simulink subsystem "Current_regulator"  (R2024b)
settings: Solver=VariableStepAuto  StartTime=0.0  StopTime=10.0  RelTol=1e-3
undefined symbols (not defined in the file): CurrentKi, CurrentKp, Ts0
libraries: simulink x1
settings Model: DataDictionary=RectData.sldd  EnableAccessToBaseWorkspace=off  Creator=sgade  LastModifiedBy=sgade

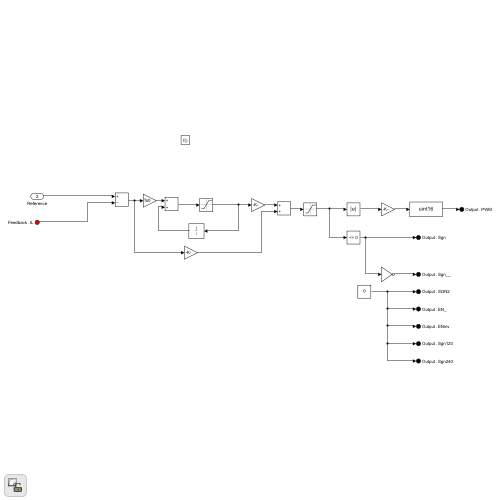
[thumbnail: Simulink's stored preview of the top-level diagram]
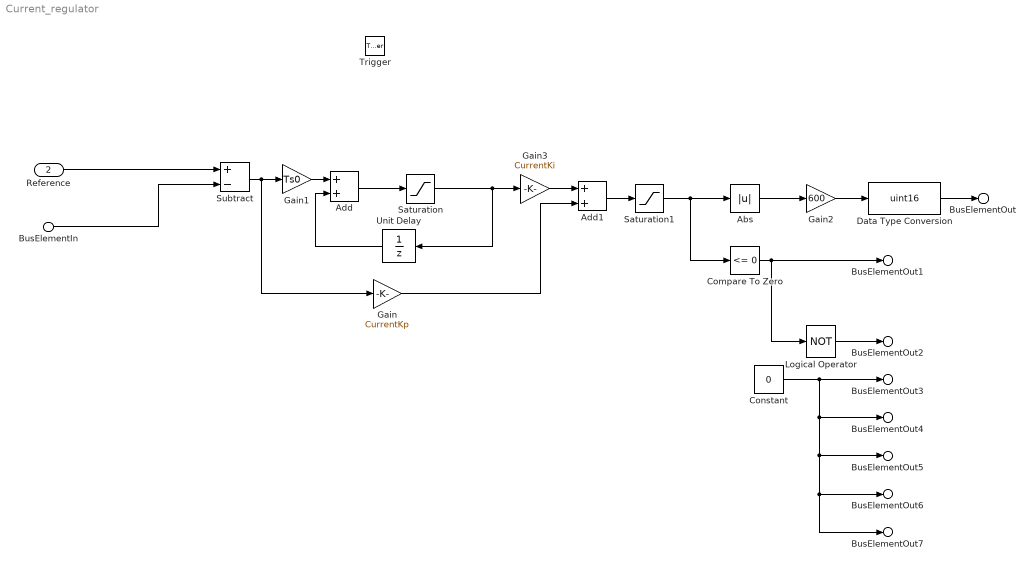
== system Current_regulator ==
  BusElementIn : Inport  PortName=Feedback  Element=IL
  Reference : Inport  Port=2
  Trigger : TriggerPort  TriggerType=function-call  VariantControl=(inherit)  PortDimensions=1
  Abs : Abs  SaturateOnIntegerOverflow=off
  Add : Sum
  Add1 : Sum
  Compare To Zero : simulink/Logic and Bit Operations/Compare To Zero  relop=<=  OutDataTypeStr=boolean
  Constant : Constant  Value=0  OutDataTypeStr=boolean  SampleTime=-1
  Data Type Conversion : DataTypeConversion  OutDataTypeStr=uint16  SaturateOnIntegerOverflow=off  RndMeth=Floor
  Gain : Gain  Gain=CurrentKp  OutDataTypeStr=single
  Gain1 : Gain  Gain=Ts0  OutDataTypeStr=single
  Gain2 : Gain  Gain=600  ParamDataTypeStr=single  OutDataTypeStr=single
  Gain3 : Gain  Gain=CurrentKi  OutDataTypeStr=single
  Logical Operator : Logic  Operator=NOT  IconShape=distinctive  AllPortsSameDT=off  OutDataTypeStr=boolean
  Saturation : Saturate  UpperLimit=1  LowerLimit=-1
  Saturation1 : Saturate  UpperLimit=0.9  LowerLimit=-0.9
  Subtract : Sum  Inputs=+-
  Unit Delay : UnitDelay  SampleTime=-1  HasFrameUpgradeWarning=on
  BusElementOut : Outport  Description=PWM1-AB  PortName=Output  Element=PWM
  BusElementOut1 : Outport  Description=GPIO4  PortName=Output  Element=Sgn
  BusElementOut2 : Outport  Description=GPIO5  PortName=Output  Element=Sgn__
  BusElementOut6 : Outport  Description=GPIO22  PortName=Output  Element=Sgn120
  BusElementOut7 : Outport  Description=GPIO11  PortName=Output  Element=Sgn240
  BusElementOut4 : Outport  Description=GPIO12  PortName=Output  Element=EN_
  BusElementOut5 : Outport  Description=GPIO13  PortName=Output  Element=ENinv
  BusElementOut3 : Outport  Description=GPIO7  PortName=Output  Element=SGN2
  wires:
  Reference/1 -> Subtract/1
  BusElementIn/1 -> Subtract/2
  Add/1 -> Saturation/1
  Subtract/1 -> Gain/1, Gain1/1
  Unit Delay/1 -> Add/2
  Gain/1 -> Add1/2
  Saturation1/1 -> Abs/1, Compare To Zero/1
  Abs/1 -> Gain2/1
  Compare To Zero/1 -> Logical Operator/1, BusElementOut1/1
  Gain2/1 -> Data Type Conversion/1
  Logical Operator/1 -> BusElementOut2/1
  Data Type Conversion/1 -> BusElementOut/1
  Constant/1 -> BusElementOut3/1, BusElementOut4/1, BusElementOut5/1, BusElementOut6/1, BusElementOut7/1
  Gain1/1 -> Add/1
  Gain3/1 -> Add1/1
  Add1/1 -> Saturation1/1
  Saturation/1 -> Unit Delay/1, Gain3/1
